simulink model "code_converters"  (R2025b)
settings: Solver=VariableStepAuto  StartTime=0.0  StopTime=10.0  RelTol=1e-3
settings Model: Creator=Johan  LastModifiedBy=Johan

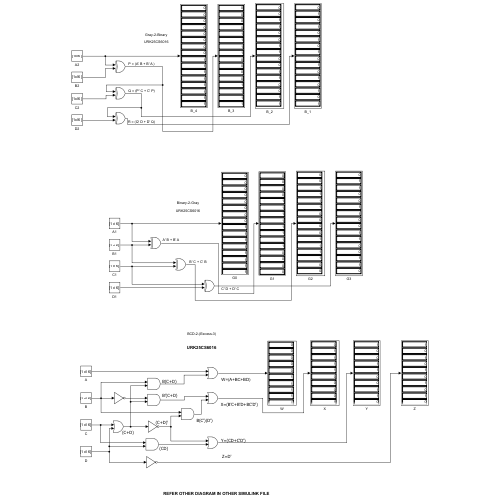
[thumbnail: Simulink's stored preview of the top-level diagram]
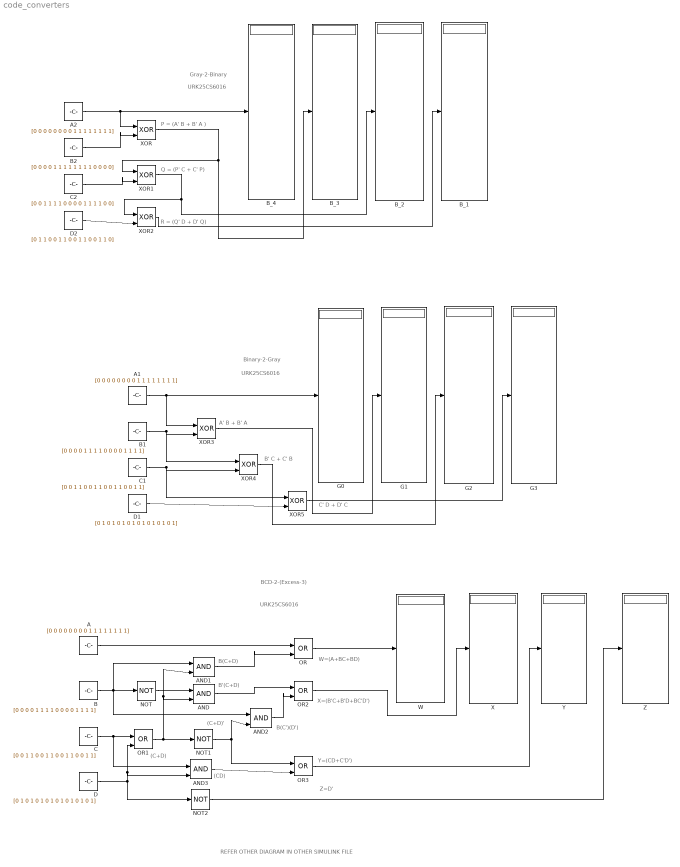
== system code_converters ==
  note: A' B + B' A
  note: W=(A+BC+BD)
  note: URK25CS6016
  note: Binary-2-Gray
  note: Gray-2-Binary
  note: URK25CS6016
  note: B(C+D)
  note: B'(C+D)
  note: X=(B'C+B'D+BC'D')
  note: Y=(CD+C'D')
  note: Z=D'
  note: (C+D)
  note: (C+D)'
  note: B(C')(D')
  note: (CD)
  note: URK25CS6016
  note: BCD-2-(Excess-3)
  note: REFER OTHER DIAGRAM IN OTHER SIMULINK FILE
  note: B' C + C' B
  note: C' D + D' C
  note: P = (A' B + B' A )
  note: Q = (P' C + C' P)
  note: R = (Q' D + D' Q)
  A : Constant  Value=[0 0 0 0 0 0 0 0 1 1 1 1 1 1 1 1]
  A1 : Constant  Value=[0 0 0 0 0 0 0 0 1 1 1 1 1 1 1 1]
  A2 : Constant  Value=[0 0 0 0 0 0 0 0 1 1 1 1 1 1 1 1]
  AND{,1..3} (4 alike) : Logic  IconShape=distinctive  AllPortsSameDT=off  OutDataTypeStr=boolean
  B : Constant  Value=[0 0 0 0 1 1 1 1 0 0 0 0 1 1 1 1]
  B1 : Constant  Value=[0 0 0 0 1 1 1 1 0 0 0 0 1 1 1 1]
  B2 : Constant  Value=[0 0 0 0 1 1 1 1 1 1 1 1 0 0 0 0]
  B_{1..4} (4 alike) : Display
  C : Constant  Value=[0 0 1 1 0 0 1 1 0 0 1 1 0 0 1 1]
  C1 : Constant  Value=[0 0 1 1 0 0 1 1 0 0 1 1 0 0 1 1]
  C2 : Constant  Value=[0 0 1 1 1 1 0 0 0 0 1 1 1 1 0 0]
  D : Constant  Value=[0 1 0 1 0 1 0 1 0 1 0 1 0 1 0 1]
  D1 : Constant  Value=[0 1 0 1 0 1 0 1 0 1 0 1 0 1 0 1]
  D2 : Constant  Value=[0 1 1 0 0 1 1 0 0 1 1 0 0 1 1 0]
  G{0..3} (4 alike) : Display
  NOT : Logic  Operator=NOT  IconShape=distinctive  AllPortsSameDT=off  OutDataTypeStr=boolean
  NOT1 : Logic  Operator=NOT  IconShape=distinctive  AllPortsSameDT=off  OutDataTypeStr=boolean
  NOT2 : Logic  Operator=NOT  IconShape=distinctive  AllPortsSameDT=off  OutDataTypeStr=boolean
  OR{,1..3} (4 alike) : Logic  Operator=OR  IconShape=distinctive  AllPortsSameDT=off  OutDataTypeStr=boolean
  W : Display
  X : Display
  XOR{,1..5} (6 alike) : Logic  Operator=XOR  IconShape=distinctive  AllPortsSameDT=off  OutDataTypeStr=boolean
  Y : Display
  Z : Display
  wires:
  A2/1 -> B_4/1, XOR/1
  B2/1 -> XOR/2
  XOR/1 -> XOR1/1, B_3/1
  XOR1/1 -> B_2/1, XOR2/1
  D2/1 -> XOR2/2
  XOR2/1 -> B_1/1
  A1/1 -> G0/1, XOR3/1
  B1/1 -> XOR3/2, XOR4/1
  C1/1 -> XOR4/2, XOR5/1
  D1/1 -> XOR5/2
  XOR3/1 -> G1/1
  XOR4/1 -> G2/1
  XOR5/1 -> G3/1
  A/1 -> OR/1
  B/1 -> AND2/1, AND1/1, NOT/1
  NOT/1 -> AND/1
  OR1/1 -> AND1/2, AND/2, NOT1/1
  NOT1/1 -> OR3/1, AND2/2
  D/1 -> NOT2/1, AND3/2, OR1/2
  AND1/1 -> OR/2
  AND/1 -> OR2/1
  AND2/1 -> OR2/2
  C/1 -> AND3/1, OR1/1
  OR2/1 -> X/1
  AND3/1 -> OR3/2
  OR/1 -> W/1
  OR3/1 -> Y/1
  NOT2/1 -> Z/1
  C2/1 -> XOR1/2
